simulink model "HW_P3_8_2"  (R2014a)
settings: Solver=ode45  StartTime=0.0  StopTime=3  RelTol=1e-3
settings Model: Creator=pengpeng  LastModifiedBy=pengpeng

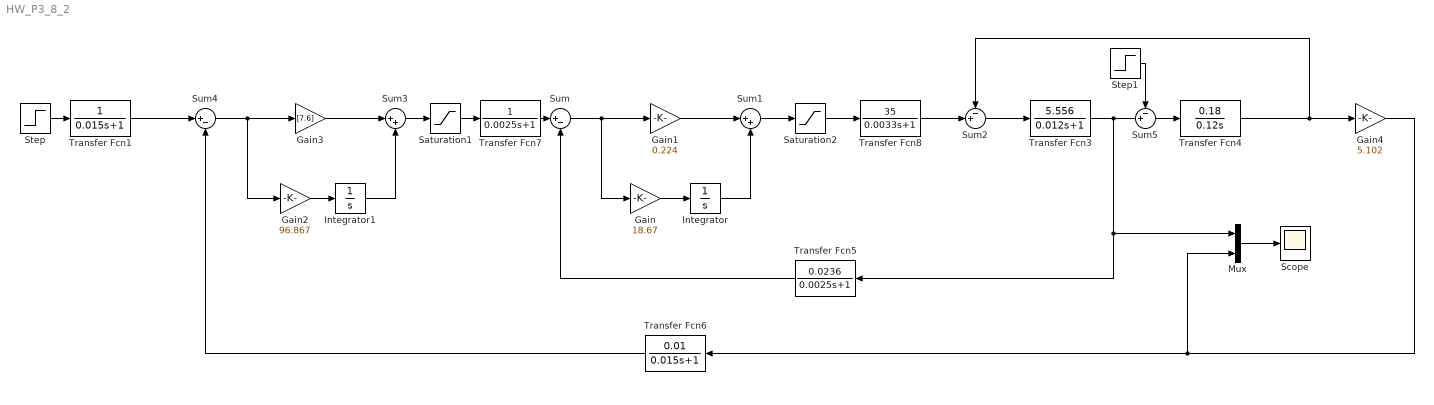
== system HW_P3_8_2 ==
  Gain : Gain  Gain=18.67
  Gain1 : Gain  Gain=0.224
  Gain2 : Gain  Gain=96.867
  Gain3 : Gain  Gain=[7.6]
  Gain4 : Gain  Gain=5.102
  Integrator : Integrator  LimitOutput=on  UpperSaturationLimit=10  LowerSaturationLimit=-10
  Integrator1 : Integrator  LimitOutput=on  UpperSaturationLimit=10  LowerSaturationLimit=-10
  Mux : Mux  Inputs=2
  Saturation1 : Saturate  UpperLimit=10  LowerLimit=-10
  Saturation2 : Saturate  UpperLimit=10  LowerLimit=-10
  Scope : Scope
      settings: TimeRange=2
  Step : Step  Before=10  After=10  SampleTime=0
  Step1 : Step  Before=10  After=0  SampleTime=0
  Sum : Sum  Inputs=|+-
  Sum1 : Sum  Inputs=|++
  Sum2 : Sum  Inputs=-+|
  Sum3 : Sum  Inputs=|++
  Sum4 : Sum  Inputs=|+-
  Sum5 : Sum  Inputs=-+|
  Transfer Fcn1 : TransferFcn  Denominator=[0.015 1]
  Transfer Fcn3 : TransferFcn  Numerator=[5.556]  Denominator=[0.012 1]
  Transfer Fcn4 : TransferFcn  Numerator=[0.18]  Denominator=[0.12 0]
  Transfer Fcn5 : TransferFcn  Numerator=[0.0236]  Denominator=[0.0025 1]
  Transfer Fcn6 : TransferFcn  Numerator=[0.01]  Denominator=[0.015 1]
  Transfer Fcn7 : TransferFcn  Denominator=[0.0025 1]
  Transfer Fcn8 : TransferFcn  Numerator=[35]  Denominator=[0.0033 1]
  wires:
  Transfer Fcn7/1 -> Sum/1
  Sum/1 -> Gain1/1, Gain/1
  Gain/1 -> Integrator/1
  Gain1/1 -> Sum1/1
  Integrator/1 -> Sum1/2
  Transfer Fcn8/1 -> Sum2/2
  Sum2/1 -> Transfer Fcn3/1
  Sum1/1 -> Saturation2/1
  Transfer Fcn4/1 -> Gain4/1, Sum2/1
  Transfer Fcn5/1 -> Sum/2
  Gain2/1 -> Integrator1/1
  Gain3/1 -> Sum3/1
  Integrator1/1 -> Sum3/2
  Step/1 -> Transfer Fcn1/1
  Transfer Fcn1/1 -> Sum4/1
  Transfer Fcn6/1 -> Sum4/2
  Sum4/1 -> Gain2/1, Gain3/1
  Transfer Fcn3/1 -> Transfer Fcn4/1, Transfer Fcn5/1, Mux/1
  Gain4/1 -> Mux/2, Transfer Fcn6/1
  Sum3/1 -> Saturation1/1
  Mux/1 -> Scope/1
  Saturation1/1 -> Transfer Fcn7/1
  Saturation2/1 -> Transfer Fcn8/1
  Step1/1 -> Sum5/1
